simulink model "mariner_sim"  (R2018b)
settings: Solver=ode1  StartTime=0.0  StopTime=600  FixedStep=0.1  RelTol=1e-3
libraries: neural x408, simulink x2
(part 22 of 22)

== system mariner_sim/Plant/NN plant mariner (No delta_dot)/Layer 6/Delays 1 ==
  "p{6}" : Inport  PortDimensions=24
      mask Display: e = 0.06;c1 = [120 230 180]/255;c2 = ([120 230 180]+0)/(256+128);c3 = ([120 230 180]+128)/(256+128);patch([0 1 1 0],[0 0 1 1],c1);patch([0 1 1 1-e 1-e 0+e],[0 0 1 1-e 0+e 0+e],c2);patch([0 0 1 1-e 0+e 0+e],[0 1 1 1-e 1-e 0+e],c3);plot([0 1 1 0 0],[0 0 1 1 0]);
  mux : Mux  Inputs=1
      mask Display: e = 0.06;c1 = [120 150 230]/255;c2 = ([120 150 230]+0)/383;c3 = ([120 150 230]+128)/383;patch([0 1 1 0],[0 0 1 1],c1);patch([0 1 1 1-e 1-e 0+e],[0 0 1 1-e 0+e 0+e],c2);patch([0 0 1 1-e 0+e 0+e],[0 1 1 1-e 1-e 0+e],c3);plot([0 1 1 0 0],[0 0 1 1 0]);disp('Mux')
  "pd{6,5}" : Outport
      mask Display: e = 0.06;c1 = [120 230 180]/255;c2 = ([120 230 180]+0)/(256+128);c3 = ([120 230 180]+128)/(256+128);patch([0 1 1 0],[0 0 1 1],c1);patch([0 1 1 1-e 1-e 0+e],[0 0 1 1-e 0+e 0+e],c2);patch([0 0 1 1-e 0+e 0+e],[0 1 1 1-e 1-e 0+e],c3);plot([0 1 1 0 0],[0 0 1 1 0]);
  wires:
  mux/1 -> "pd{6,5}"/1
  "p{6}"/1 -> mux/1

== system mariner_sim/Plant/NN plant mariner (No delta_dot)/Layer 6/LW{6,5} ==
  "ad{6,5}" : Inport  PortDimensions=24
      mask Display: e = 0.06;c1 = [120 230 180]/255;c2 = ([120 230 180]+0)/(256+128);c3 = ([120 230 180]+128)/(256+128);patch([0 1 1 0],[0 0 1 1],c1);patch([0 1 1 1-e 1-e 0+e],[0 0 1 1-e 0+e 0+e],c2);patch([0 0 1 1-e 0+e 0+e],[0 1 1 1-e 1-e 0+e],c3);plot([0 1 1 0 0],[0 0 1 1 0]);
  "IW{6,5}(1,:)'" : Constant  Value=[3.2433598998004699938586814500496302571264095604419708251953125e-05;-0.00021746891264327707147911705742870935864630155265331268310546875;-6.2519957775104847519202777572644436077098362147808074951171875e-05;-0.0002151214461402426174514712631236079687369056046009063720703125;-7.72914603333618179491215638421408584690652787685394287109375e-05;9.8220947618367704444290733345468424886348657310009002685546875e-05;0.0001382930564768189885156701723900596334715373814105987548828125;0.0001645748510074347280458806341840727327507920563220977783203125;0.000268939822215103450930850925715276389382779598236083984375;6.2985224591444543651257148564326371342758648097515106201171875e-05;5.6838608479464312821347223014800675855440204031765460968017578125e-06;2.01845702968149283613487343647108218647190369665622711181640625e-05;0.0001676190564912218385930364750180388000444509088993072509765625;0.000135878965702839718705796645537020594929344952106475830078125;6.2205662182553546173113812045585291343741118907928466796875e-05;0.000111446864397163089934784940826517640743986703455448150634765625;-5.8634943766458073424502513149025872962738503701984882354736328125e-06;0.000112997310599974860162962586596080427625565789639949798583984375;2.846586362506669975656024840215962967704399488866329193115234375e-05;-0.0001710958953371501914571262137343410358880646526813507080078125;2.73394004824882604748857717336107953087775968015193939208984375e-05;-6.170901822294167123061914281834106077440083026885986328125e-05;8.1478519128559822736097839612767756989342160522937774658203125e-05;4.553422019458672740689630931143483394407667219638824462890625e-05]
      mask Display: e = 0.06;c1 = [120 150 230]/255;c2 = ([120 150 230]+0)/383;c3 = ([120 150 230]+128)/383;patch([0 1 1 0],[0 0 1 1],c1);patch([0 1 1 1-e 1-e 0+e],[0 0 1 1-e 0+e 0+e],c2);patch([0 0 1 1-e 0+e 0+e],[0 1 1 1-e 1-e 0+e],c3);plot([0 1 1 0 0],[0 0 1 1 0]);disp('weights');
  "IW{6,5}(2,:)'" : Constant  Value=[-0.000826529499500064574780966442091312273987568914890289306640625;-0.000642491212784880995172176465501934217172674834728240966796875;-0.00089601761422035386926709943367086452781222760677337646484375;0.0003640521562445046019167171902353175028110854327678680419921875;-0.0022597717662539919432351798178615354117937386035919189453125;-5.95161806487568421550858610569179063531919382512569427490234375e-05;-0.00025641552490142881758072856968055930337868630886077880859375;0.00080747921980977373397625473927519124117679893970489501953125;-0.00042040003190180522639474158808070569648407399654388427734375;0.0018262459479417773693110671473505135509185492992401123046875;-0.00146586650901986935424670122074530809186398983001708984375;7.8763674807919793123371643428498600769671611487865447998046875e-05;-0.00010991751878111353829710339358172177526284940540790557861328125;-0.00036678182453456676000158598327516301651485264301300048828125;-0.0003171821049869377631517941562577789227361790835857391357421875;0.000251068945369483233036322911146953629213385283946990966796875;-0.001212130785092036151795458209790012915618717670440673828125;0.000947577323859999267989528970446144739980809390544891357421875;0.00052599882450631301085419710972246321034617722034454345703125;-0.00081217642806952791527386192882431714679114520549774169921875;0.0047275051808355512961146160932912607677280902862548828125;-0.000635378248235334550965414113221640945994295179843902587890625;9.64182414439658107448150037299683390301652252674102783203125e-05;0.0001731850016870155610677894930660158934188075363636016845703125]
      mask Display: e = 0.06;c1 = [120 150 230]/255;c2 = ([120 150 230]+0)/383;c3 = ([120 150 230]+128)/383;patch([0 1 1 0],[0 0 1 1],c1);patch([0 1 1 1-e 1-e 0+e],[0 0 1 1-e 0+e 0+e],c2);patch([0 0 1 1-e 0+e 0+e],[0 1 1 1-e 1-e 0+e],c3);plot([0 1 1 0 0],[0 0 1 1 0]);disp('weights');
  "IW{6,5}(3,:)'" : Constant  Value=[2.46152644631382654040636925873997142844018526375293731689453125e-05;-2.563158103268046409013714015401319556985981762409210205078125e-05;1.19444456304550761520551216410268580148112960159778594970703125e-05;-3.8165061632398022094248002389349494478665292263031005859375e-05;3.2095720426049420353174779219074252978316508233547210693359375e-05;2.005335334908526424726842030121787274765665642917156219482421875e-05;4.76339293072544701685040735572584935653139837086200714111328125e-05;1.7604738734322618212528588355070269244606606662273406982421875e-05;6.1921630995887057030864497608746432888437993824481964111328125e-05;-2.677483879698117457388885365165975827039801515638828277587890625e-05;2.65402830536713558421020586752803183117066510021686553955078125e-05;6.980146402722020059004696956872493274204316549003124237060546875e-06;4.91862369857580910268747553804047356607043184340000152587890625e-05;9.398121921791441398127096851222717077689594589173793792724609375e-06;2.849932108961100444741686155136761726680560968816280364990234375e-05;2.474611348555533069906893495204514010765706188976764678955078125e-05;3.89805031900851425646047088147128079071990214288234710693359375e-05;-7.06469847394216254009291500182143863639794290065765380859375e-07;1.40147477682385900184768023901682454379624687135219573974609375e-05;-9.1741821131806661920350676187041472076089121401309967041015625e-06;-0.00012599257486806556753482222443807359013590030372142791748046875;7.964410532433889255391097627967411654026363976299762725830078125e-06;2.9571704172556262228167833772118910928838886320590972900390625e-05;-5.5995289024227002996621053998449468735998379997909069061279296875e-06]
      mask Display: e = 0.06;c1 = [120 150 230]/255;c2 = ([120 150 230]+0)/383;c3 = ([120 150 230]+128)/383;patch([0 1 1 0],[0 0 1 1],c1);patch([0 1 1 1-e 1-e 0+e],[0 0 1 1-e 0+e 0+e],c2);patch([0 0 1 1-e 0+e 0+e],[0 1 1 1-e 1-e 0+e],c3);plot([0 1 1 0 0],[0 0 1 1 0]);disp('weights');
  "IW{6,5}(4,:)'" : Constant  Value=[-0.1046999224485727630895581796721671707928180694580078125;-0.214859862140896529236755441161221824586391448974609375;-0.11414394274893570335738246512846671976149082183837890625;-0.193735966562724792883187774350517429411411285400390625;-0.1777661283319564855531780267483554780483245849609375;-0.406317254503526459341600229890900664031505584716796875;0.09130499074981761331581964213910396210849285125732421875;-0.08355202175896110639019553900652681477367877960205078125;0.004607169690688232670250368272490959498099982738494873046875;0.11331833976123040219619042545673437416553497314453125;0.12349327484238233065827472501041484065353870391845703125;-0.09737098152361088609918482461580424569547176361083984375;-0.172392956306251454723366123289451934397220611572265625;-0.05354406813646846174936655415876884944736957550048828125;0.0788347063873013897961072871112264692783355712890625;0.131548859513590021830253817824996076524257659912109375;0.258288818657371466169792029177187941968441009521484375;-0.3513774626571934955876486128545366227626800537109375;0.1285503858247094288724809985069441609084606170654296875;0.1822954729789078853752215536587755195796489715576171875;-0.05059362603293506011059577076593996025621891021728515625;0.1611838123398981748035652117323479615151882171630859375;-0.001358270969995178760469922707443402032367885112762451171875;0.1691231424475345967994854845528607256710529327392578125]
      mask Display: e = 0.06;c1 = [120 150 230]/255;c2 = ([120 150 230]+0)/383;c3 = ([120 150 230]+128)/383;patch([0 1 1 0],[0 0 1 1],c1);patch([0 1 1 1-e 1-e 0+e],[0 0 1 1-e 0+e 0+e],c2);patch([0 0 1 1-e 0+e 0+e],[0 1 1 1-e 1-e 0+e],c3);plot([0 1 1 0 0],[0 0 1 1 0]);disp('weights');
  "IW{6,5}(5,:)'" : Constant  Value=[-0.261050291944736445604036134682246483862400054931640625;0.21688530390838633987726780105731450021266937255859375;-0.0263686731508492311348845760221593081951141357421875;-0.0783502653405710181022669758021947927772998809814453125;-0.0574573045503896373542573883241857402026653289794921875;-0.02833691747677068162314384380806586705148220062255859375;0.306787389727579518083899756675236858427524566650390625;0.4115796583411033271460155447130091488361358642578125;-0.0884904419428817756720917486745747737586498260498046875;-0.04625755795249515689437913579240557737648487091064453125;-0.01312950851618376220397710341103447717614471912384033203125;0.148726783593528200100308822584338486194610595703125;-0.24354178610612653432809793230262584984302520751953125;0.2624174384097830436957110578077845275402069091796875;0.480136430526202584445627508102916181087493896484375;-0.3441908584282888927674548540380783379077911376953125;-0.145810822380717741708622270380146801471710205078125;0.307466536601382178783836707225418649613857269287109375;-0.1708275816058468787872470784350298345088958740234375;-0.22206736034940333102127851816476322710514068603515625;0.05136313987499152577953509535291232168674468994140625;0.0226850580484755093291227012741728685796260833740234375;-0.50394671901843557382250082810060121119022369384765625;-0.1788429832334376412550369650489301420748233795166015625]
      mask Display: e = 0.06;c1 = [120 150 230]/255;c2 = ([120 150 230]+0)/383;c3 = ([120 150 230]+128)/383;patch([0 1 1 0],[0 0 1 1],c1);patch([0 1 1 1-e 1-e 0+e],[0 0 1 1-e 0+e 0+e],c2);patch([0 0 1 1-e 0+e 0+e],[0 1 1 1-e 1-e 0+e],c3);plot([0 1 1 0 0],[0 0 1 1 0]);disp('weights');
  "IW{6,5}(6,:)'" : Constant  Value=[-8.3873490168356670273162867257354946559644304215908050537109375e-05;0.00147502001895182498214520450119380257092416286468505859375;0.000330261437779736277860209714418715520878322422504425048828125;0.00133625764264578878078026935583011436392553150653839111328125;0.00085914790987545578727913042627051254385150969028472900390625;-0.000567433998010235108970522599491914661484770476818084716796875;-0.0010907273517562336186126348280822639935649931430816650390625;-0.00133779757933903263762698276906348837655968964099884033203125;-0.00234554091843410493500865499072460806928575038909912109375;-0.0001144305367251422498632573709897997105144895613193511962890625;0.0003636845135138208986481933582268766258493997156620025634765625;-2.0497064683987363986790442016427959970314987003803253173828125e-05;-0.0013673893877836052444807446448749033152125775814056396484375;-0.00079367129654968858465391434720004326663911342620849609375;-0.000418521036158354671312398220806016979622654616832733154296875;-0.00104356258505614442159969978973776960629038512706756591796875;-0.000101142753841237495091541498393183928783400915563106536865234375;-0.00091411335818792249958975038026665060897357761859893798828125;-0.000743367293182789989035297306685379226109944283962249755859375;0.000889863084029751433452759545872368107666261494159698486328125;0.000803295392184018319271798791447736221016384661197662353515625;0.0004381772186861732716785244878821004022029228508472442626953125;-0.00147945223686744516990165809744439684436656534671783447265625;-0.0002851975628954128987209426515647692212951369583606719970703125]
      mask Display: e = 0.06;c1 = [120 150 230]/255;c2 = ([120 150 230]+0)/383;c3 = ([120 150 230]+128)/383;patch([0 1 1 0],[0 0 1 1],c1);patch([0 1 1 1-e 1-e 0+e],[0 0 1 1-e 0+e 0+e],c2);patch([0 0 1 1-e 0+e 0+e],[0 1 1 1-e 1-e 0+e],c3);plot([0 1 1 0 0],[0 0 1 1 0]);disp('weights');
  Mux : Mux  Inputs=6
      mask Display: e = 0.06;c1 = [120 150 230]/255;c2 = ([120 150 230]+0)/383;c3 = ([120 150 230]+128)/383;patch([0 1 1 0],[0 0 1 1],c1);patch([0 1 1 1-e 1-e 0+e],[0 0 1 1-e 0+e 0+e],c2);patch([0 0 1 1-e 0+e 0+e],[0 1 1 1-e 1-e 0+e],c3);plot([0 1 1 0 0],[0 0 1 1 0]);disp('Mux');
  dotprod{1..6} (6 alike) : neural/Weight Functions/dotprod
  "lz{6,5}" : Outport
      mask Display: e = 0.06;c1 = [120 230 180]/255;c2 = ([120 230 180]+0)/(256+128);c3 = ([120 230 180]+128)/(256+128);patch([0 1 1 0],[0 0 1 1],c1);patch([0 1 1 1-e 1-e 0+e],[0 0 1 1-e 0+e 0+e],c2);patch([0 0 1 1-e 0+e 0+e],[0 1 1 1-e 1-e 0+e],c3);plot([0 1 1 0 0],[0 0 1 1 0]);
  wires:
  Mux/1 -> "lz{6,5}"/1
  dotprod6/1 -> Mux/6
  "IW{6,5}(6,:)'"/1 -> dotprod6/1
  dotprod5/1 -> Mux/5
  "IW{6,5}(5,:)'"/1 -> dotprod5/1
  dotprod4/1 -> Mux/4
  "IW{6,5}(4,:)'"/1 -> dotprod4/1
  dotprod3/1 -> Mux/3
  "IW{6,5}(3,:)'"/1 -> dotprod3/1
  dotprod2/1 -> Mux/2
  "IW{6,5}(2,:)'"/1 -> dotprod2/1
  dotprod1/1 -> Mux/1
  "ad{6,5}"/1 -> dotprod6/2, dotprod5/2, dotprod4/2, dotprod3/2, dotprod2/2, dotprod1/2
  "IW{6,5}(1,:)'"/1 -> dotprod1/1

== matlab function mariner_sim/MATLAB Function1 ==
  data: xdot input; xnext output; x input; h input
function xnext = euler2(xdot,x,h)
% EULER2  Integrate a system of ordinary differential equations using 
%	  Euler's 2nd-order method.
%
% xnext = euler2(xdot,x,h)
%
% xdot  - dx/dt(k) = f(x(k)
% x     - x(k)
% xnext - x(k+1)
% h     - step size
%
% Author:   Thor I. Fossen
% Date:     14th June 2001
% Revisions: 

xnext = x + h*xdot;

== matlab function mariner_sim/MATLAB Function ==
  data: x input; xdot output; ui input
function xdot   = mariner(x,ui)
% [xdot,U] = mariner(x,ui) returns the speed U in m/s (optionally) and the 
% time derivative of the state vector: x = [ u v r x y psi delta n ]'  for
% the Mariner class vessel L = 160.93 m, where
%
% u     = pertubed surge velocity about Uo (m/s)
% v     = pertubed sway velocity about zero (m/s)
% r     = pertubed yaw velocity about zero (rad/s)
% x     = position in x-direction (m)
% y     = position in y-direction (m)
% psi   = pertubed yaw angle about zero (rad)
% delta = actual rudder angle (rad)
%
% The inputs are :
% 
% ui    = commanded rudder angle (rad)
% U0    = nominal speed (optionally). Default value is U0 = 7.7175 m/s = 15 knots.
%
% Reference: M.S. Chislett and J. Stroem-Tejsen (1965). Planar Motion Mechanism Tests 
%            and Full-Scale Steering and Maneuvering Predictions for a Mariner Class Vessel,
%            Technical Report Hy-5, Hydro- and Aerodynamics Laboratory, Lyngby, Denmark.
% 
% Author:    Trygve Lauvdal
% Date:      12th May 1994
% Revisions: 19th July 2001 (Thor I. Fossen): added input/ouput U0 and U, changed order of x-vector
%            20th July 2001 (Thor I. Fossen): replaced inertia matrix with correct values
%            11th July 2003 (Thor I. Fossen): max rudder is changed from 30 deg to 40
%                            deg to satisfy IMO regulations for 35 deg rudder execute

% Check of input and state dimensions
if (length(x)  ~= 7),error('x-vector must have dimension 7 !'); end
if (length(ui) ~= 1),error('ui must be a scalar input!'); end
%if nargin==2, U0 = 7.7175; end

U0 = 7.7175;

% Normalization variables
L = 160.93;
U = sqrt((U0 + x(1))^2 + x(2)^2);

% Non-dimensional states and inputs
delta_c = -ui;   % delta_c = -ui such that positive delta_c -> positive r

u     = x(1)/U;   
v     = x(2)/U;  
r     = x(3)*L/U; 
psi   = x(6); 
delta = x(7); 

% Parameters, hydrodynamic derivatives and main dimensions
delta_max  = 40;           % max rudder angle      (deg)
Ddelta_max = 5;            % max rudder derivative (deg/s)

m  = 798e-5;
Iz = 39.2e-5;
xG = -0.023;

Xudot =  -42e-5;   Yvdot =  -748e-5;   Nvdot = 4.646e-5;
Xu    = -184e-5;   Yrdot =-9.354e-5;   Nrdot = -43.8e-5;
Xuu   = -110e-5;   Yv    = -1160e-5;   Nv    =  -264e-5;
Xuuu  = -215e-5;   Yr    =  -499e-5;   Nr    =  -166e-5;
Xvv   = -899e-5;   Yvvv  = -8078e-5;   Nvvv  =  1636e-5;
Xrr   =   18e-5;   Yvvr  = 15356e-5;   Nvvr  = -5483e-5;
Xdd   =  -95e-5;   Yvu   = -1160e-5;   Nvu   =  -264e-5;
Xudd  = -190e-5;   Yru   =  -499e-5;   Nru   =  -166e-5;
Xrv   =  798e-5;   Yd    =   278e-5;   Nd    =  -139e-5;
Xvd   =   93e-5;   Yddd  =   -90e-5;   Nddd  =    45e-5;
Xuvd  =   93e-5;   Yud   =   556e-5;   Nud   =  -278e-5;
                   Yuud  =   278e-5;   Nuud  =  -139e-5;
                   Yvdd  =    -4e-5;   Nvdd  =    13e-5;
                   Yvvd  =  1190e-5;   Nvvd  =  -489e-5;
                   Y0    =    -4e-5;   N0    =     3e-5;
                   Y0u   =    -8e-5;   N0u   =     6e-5;
                   Y0uu  =    -4e-5;   N0uu  =     3e-5;

% Masses and moments of inertia
m11 = m-Xudot;
m22 = m-Yvdot;
m23 = m*xG-Yrdot;
m32 = m*xG-Nvdot;
m33 = Iz-Nrdot;

% Rudder saturation and dynamics
if abs(delta_c) >= delta_max*pi/180,
   delta_c = sign(delta_c)*delta_max*pi/180;
end
delta_dot = delta_c - delta;
if abs(delta_dot) >= Ddelta_max*pi/180,
   delta_dot = sign(delta_dot)*Ddelta_max*pi/180;
end

% Forces and moments
X = Xu*u + Xuu*u^2 + Xuuu*u^3 + Xvv*v^2 + Xrr*r^2 + Xrv*r*v + Xdd*delta^2 +...
    Xudd*u*delta^2 + Xvd*v*delta + Xuvd*u*v*delta;

Y = Yv*v + Yr*r + Yvvv*v^3 + Yvvr*v^2*r + Yvu*v*u + Yru*r*u + Yd*delta + ...
    Yddd*delta^3 + Yud*u*delta + Yuud*u^2*delta + Yvdd*v*delta^2 + ...
    Yvvd*v^2*delta + (Y0 + Y0u*u + Y0uu*u^2);

N = Nv*v + Nr*r + Nvvv*v^3 + Nvvr*v^2*r + Nvu*v*u + Nru*r*u + Nd*delta + ...
    Nddd*delta^3 + Nud*u*delta + Nuud*u^2*delta + Nvdd*v*delta^2 + ...
    Nvvd*v^2*delta + (N0 + N0u*u + N0uu*u^2);

% Dimensional state derivative
detM22 = m22*m33-m23*m32;

xdot = [           X*(U^2/L)/m11
        -(-m33*Y+m23*N)*(U^2/L)/detM22
         (-m32*Y+m22*N)*(U^2/L^2)/detM22
           (cos(psi)*(U0/U+u)-sin(psi)*v)*U
           (sin(psi)*(U0/U+u)+cos(psi)*v)*U  
                    r*(U/L)
                    delta_dot                  ];

== stateflow chart mariner_sim/mariner ==
  settings: updateMethod=CONTINUOUS
  state mariner
    %% initialize values when entry
    en:
    L = 160.93;
    m = 798*10^-5;
    xG = -0.023;
    Iz = 39.2*10^-5;
    Xudot =  -42e-5;  Yvdot =  -748e-5;  Nvdot = 4.646e-5;
    Xu  = -184e-5;   Yrdot =-9.354e-5;   Nrdot = -43.8e-5;
    Xuu = -110e-5;   Yv = -1160e-5;   Nv =  -264e-5;
    Xuuu = -215e-5;   Yr =  -499e-5;   Nr =  -166e-5;
    Xvv = -899e-5;   Yvvv = -8078e-5;   Nvvv =  1636e-5;
    Xrr =   18e-5;   Yvvr = 15356e-5;   Nvvr = -5483e-5;
    Xdd =  -95e-5;   Yvu = -1160e-5;   Nvu =  -264e-5;
    Xudd = -190e-5;   Yru =  -499e-5;   Nru =  -166e-5;
    Xrv =  798e-5;   Yd  =   278e-5;   Nd =  -139e-5;
    Xvd =   93e-5;   Yddd  =   -90e-5;   Nddd =    45e-5;
    Xuvd =   93e-5;   Yud = 556e-5;   Nud =  -278e-5;
    Yuud =   278e-5;   Nuud  =  -139e-5;
    Yvdd  =    -4e-5;   Nvdd  = 13e-5;
    Yvvd  =  1190e-5;   Nvvd  = -489e-5;
    Y0 = -4e-5;   N0 =  3e-5;
    Y0u  =  -8e-5;   N0u = 6e-5;
    Y0uu =  -4e-5;   N0uu  =  3e-5;
    m11 = 798*10^-5 - (-42e-5);
    m22 = 798*10^-5 - ( -748e-5);
    m23 = 798*10^-5 * -0.023 - (-9.354e-5);
    m32 = 798*10^-5 * -0.023 - 4.646e-5;
    m33 = 39.2*10^-5 -  (-43.8e-5);
    %detM22 = m22*m33-m23*m32;
    %detM22 = ((798*10^-5 - ( -748e-5))*(39.2*10^-5 -  (-43.8e-5)) - (798*10^-5 * -0.023 - (-9.354e-5))*(798*10^-5 * -0.023 - 4.646e-5));
    delta_max = 40;
    Ddelta_max = 5;
    % u
    %Executing updates of system during simulation
    du:
    %delta_c = min(max(-ui,-delta_max*pi/180),delta_max*pi/180) ;
    %U = (sqrt((ui + u)^2 + v^2));
    %delta_do = (-ui - delta);
    %X = Xu*u/(sqrt((ui + u)^2 + v^2)) + Xuu*(u/(sqrt((ui + u)^2 + v^2)))^2 + Xuuu*(u/(sqrt((ui + u)^2 + v^2)))^3 + Xvv*(v/(sqrt((ui + u)^2 + v^2)))^2 + Xrr*(r*L/(sqrt((ui + u)^2 + v^2)))^2 + Xrv*(r*L/(sqrt((ui + u)^2 + v^2)))*(v/(sqrt((ui + u)^2 + v^2))) + Xdd*delta^2 +Xudd*(u/(sqrt((ui + u)^2 + v^2)))*delta^2 + Xvd*(v/(sqrt((ui + u)^2 + v^2)))*delta + Xuvd*(u/(sqrt((ui + u)^2 + v^2)))*(v/(sqrt((ui + u)^2 + v^2)))*delta;
    %Y = Yv*v + Yr*r + Yvvv*v^3 + Yvvr*v^2*r + Yvu*v*u + Yru*r*u + Yd*delta + Yddd*delta^3 + Yud*u*delta + Yuud*u^2*delta + Yvdd*v*delta^2 + Yvvd*v^2*delta + (Y0 + Y0u*u + Y0uu*u^2);
    %N = Nv*v + Nr*r + Nvvv*v^3 + Nvvr*v^2*r + Nvu*v*u + Nru*r*u + Nd*delta + Nddd*delta^3 + Nud*u*delta + Nuud*u^2*delta + Nvdd*v*delta^2 + Nvvd*v^2*delta + (N0 + N0u*u + N0uu*u^2);
    u_dot = (Xu*(u/(sqrt((ui + u)^2 + v^2))) + Xuu*(u/(sqrt((ui + u)^2 + v^2)))^2 + Xuuu*(u/(sqrt((ui + u)^2 + v^2)))^3 + Xvv*(v/(sqrt((ui + u)^2 + v^2)))^2 + Xrr*(r*L/(sqrt((ui + u)^2 + v^2)))^2 + Xrv*(r*L/(sqrt((ui + u)^2 + v^2)))*(v/(sqrt((ui + u)^2 + v^2))) + Xdd*delta^2 +Xudd*(u/(sqrt((ui + u)^2 + v^2)))*delta^2 + Xvd*(v/(sqrt((ui + u)^2 + v^2)))*delta + Xuvd*(u/(sqrt((ui + u)^2 + v^2)))*(v/(sqrt((ui + u)^2 + v^2)))*delta)*((sqrt((ui + u)^2 + v^2))^2 /L)/(798*10^-5 - (-42e-5));
    v_dot =  -(-(39.2*10^-5 -  (-43.8e-5))*(Yv*(v/(sqrt((ui + u)^2 + v^2))) + Yr*(r*L/(sqrt((ui + u)^2 + v^2))) + Yvvv*(v/(sqrt((ui + u)^2 + v^2)))^3 + Yvvr*(v/(sqrt((ui + u)^2 + v^2)))^2 * (r*L/(sqrt((ui + u)^2 + v^2))) + Yvu*(v/(sqrt((ui + u)^2 + v^2)))*(u/(sqrt((ui + u)^2 + v^2))) + Yru*(r*L/(sqrt((ui + u)^2 + v^2)))*(u/(sqrt((ui + u)^2 + v^2))) + Yd*delta + Yddd*delta^3 + Yud*(u/(sqrt((ui + u)^2 + v^2)))*delta + Yuud*(u/(sqrt((ui + u)^2 + v^2)))^2*delta + Yvdd*(v/(sqrt((ui + u)^2 + v^2)))*delta^2 + Yvvd*(v/(sqrt((ui + u)^2 + v^2)))^2*delta + (Y0 + Y0u*(u/(sqrt((ui + u)^2 + v^2))) + Y0uu*(u/(sqrt((ui + u)^2 + v^2)))^2))+(798*10^-5 * -0.023 - (-9.354e-5))*(Nv*(v/(sqrt((ui + u)^2 + v^2))) + Nr*(r*L/(sqrt((ui + u)^2 + v^2))) + Nvvv*(v/(sqrt((ui + u)^2 + v^2)))^3 + Nvvr*(v/(sqrt((ui + u)^2 + v^2)))^2*(r*L/(sqrt((ui + u)^2 + v^2))) + Nvu*(v/(sqrt((ui + u)^2 + v^2)))*(u/(sqrt((ui + u)^2 + v^2))) + Nru*(r*L/(sqrt((ui + u)^2 + v^2)))*(u/(sqrt((ui + u)^2 + v^2))) + Nd*delta + Nddd*delta^3 + Nud*(u/(sqrt((ui + u)^2 + v^2)))*delta + Nuud*(u/(sqrt((ui + u)^2 + v^2)))^2*delta + Nvdd*(v/(sqrt((ui + u)^2 + v^2)))*delta^2 + Nvvd*v^2*delta + (N0 + N0u*u + N0uu*u^2)))*((sqrt((ui + u)^2 + v^2))^2/L)/((798*10^-5 - ( -748e-5))*(39.2*10^-5 -  (-43.8e-5)) - (798*10^-5 * -0.023 - (-9.354e-5))*(798*10^-5 * -0.023 - 4.646e-5)) ;
    r_dot = (-(798*10^-5 * -0.023 - 4.646e-5)*(Yv*(v/(sqrt((ui + u)^2 + v^2))) + Yr*(r*L/(sqrt((ui + u)^2 + v^2))) + Yvvv*(v/(sqrt((ui + u)^2 + v^2)))^3 + Yvvr*(v/(sqrt((ui + u)^2 + v^2)))^2*(r*L/(sqrt((ui + u)^2 + v^2))) + Yvu*(v/(sqrt((ui + u)^2 + v^2)))*(u/(sqrt((ui + u)^2 + v^2))) + Yru*(r*L/(sqrt((ui + u)^2 + v^2)))*(u/(sqrt((ui + u)^2 + v^2))) + Yd*delta + Yddd*delta^3 + Yud*(u/(sqrt((ui + u)^2 + v^2)))*delta + Yuud*(u/(sqrt((ui + u)^2 + v^2)))^2*delta + Yvdd*(v/(sqrt((ui + u)^2 + v^2)))*delta^2 + Yvvd*(v/(sqrt((ui + u)^2 + v^2)))^2*delta + (Y0 + Y0u*(u/(sqrt((ui + u)^2 + v^2))) + Y0uu*(u/(sqrt((ui + u)^2 + v^2)))^2))+(798*10^-5 - ( -748e-5))*(Nv*(v/(sqrt((ui + u)^2 + v^2))) + Nr*(r*L/(sqrt((ui + u)^2 + v^2))) + Nvvv*(v/(sqrt((ui + u)^2 + v^2)))^3 + Nvvr*(v/(sqrt((ui + u)^2 + v^2)))^2*(r*L/(sqrt((ui + u)^2 + v^2))) + Nvu*(v/(sqrt((ui + u)^2 + v^2)))*(u/(sqrt((ui + u)^2 + v^2))) + Nru*(r*L/(sqrt((ui + u)^2 + v^2)))*(u/(sqrt((ui + u)^2 + v^2))) + Nd*delta + Nddd*delta^3 + Nud*(u/(sqrt((ui + u)^2 + v^2)))*delta + Nuud*(u/(sqrt((ui + u)^2 + v^2)))^2*delta + Nvdd*(v/(sqrt((ui + u)^2 + v^2)))*delta^2 + Nvvd*(v/(sqrt((ui + u)^2 + v^2)))^2*delta + (N0 + N0u*(u/(sqrt((ui + u)^2 + v^2))) + N0uu*(u/(sqrt((ui + u)^2 + v^2)))^2)))*((sqrt((ui + u)^2 + v^2))^2/L^2)/((798*10^-5 - ( -748e-5))*(39.2*10^-5 -  (-43.8e-5)) - (798*10^-5 * -0.023 - (-9.354e-5))*(798*10^-5 * -0.023 - 4.646e-5)) ;
    x_dot = (cos(psi)*(U0/(sqrt((ui + u)^2 + v^2))+(u/(sqrt((ui + u)^2 + v^2))))-sin(psi)*(v/(sqrt((ui + u)^2 + v^2))))*(sqrt((ui + u)^2 + v^2)) ;
    y_dot = (sin(psi)*(U0/(sqrt((ui + u)^2 + v^2))+(u/(sqrt((ui + u)^2 + v^2))))+cos(psi)*(v/(sqrt((ui + u)^2 + v^2))))*(sqrt((ui + u)^2 + v^2)) ;
    psi_dot = (r*L/(sqrt((ui + u)^2 + v^2)))*((sqrt((ui + u)^2 + v^2))/L);
    delta_dot = min(max(((min(max(-ui,-delta_max*pi/180),delta_max*pi/180)) - delta),-Ddelta_max*pi/180),Ddelta_max*pi/180) ;
    %% OUTPUTS
    u_out = u;
    v_out = v;
    r_out = r;
    x_out = x;
    y_out = y;
    psi_out = psi;
    delta_out = delta;
  (default) -> ? [order 1]
  (default) -> mariner [order 1] : {u = 0.01;
      | v = 0.01;
      | r = 0.01;
      | x = 0.01;
      | y = 0.01;
      | psi = 0.01;
      | delta = 0.01;}
  data: u_out output; v_out output; u local; ui input; v local; Nvdot local double; Iz local double; L local double; Yvdot local double; xG local double; m local double; Xudot local double; Xuu local double; Yv local double; Xuuu local double; Nrdot local double; Nv local double; Yr local double; Yrdot local double; Xu local double; Nr local double; Xrr local double; Xdd local double; Yvvv local double; Yvu local double; Nvvv local double; Yvvr local double; Nvvr local double; Xvv local double; Xvd local double; Yru local double; Nd local double; Nvu local double; Xudd local double; Nru local double; Yd local double; Xrv local double; Nvdd local double; Yud local double; Yuud local double; Xuvd local double; Yvdd local double; Nud local double; Nuud local double; Yddd local double; Nddd local double; Y0uu local double; N0uu local double; N0 local double; N0u local double; Y0 local double; Yvvd local double; Nvvd local double; Y0u local double; m11 local double; m32 local double; m22 local double; m23 local double; m33 local double; U0 input; r_out output; r local; psi local; x local; y local; delta local; Ddelta_max local double; delta_max local double; N local double; x_out output; y_out output; psi_out output double; delta_out output
  data u settings: updateMethod=SF_CONTINUOUS_TIME_DATA
  data v settings: updateMethod=SF_CONTINUOUS_TIME_DATA
  data r settings: updateMethod=SF_CONTINUOUS_TIME_DATA
  data psi settings: updateMethod=SF_CONTINUOUS_TIME_DATA
  data x settings: updateMethod=SF_CONTINUOUS_TIME_DATA
  data y settings: updateMethod=SF_CONTINUOUS_TIME_DATA
  data delta settings: updateMethod=SF_CONTINUOUS_TIME_DATA

== matlab function mariner_sim/Plant/delta_dot ==
  data: u input; y output
function y = fcn(u)

% Parameters, hydrodynamic derivatives and main dimensions
delta_max  = 40;           % max rudder angle      (deg)
Ddelta_max = 5;            % max rudder derivative (deg/s)

% Non-dimensional states and inputs
delta_c = -u(8);   % delta_c = -ui such that positive delta_c -> positive 

% Rudder saturation and dynamics
if abs(delta_c) >= delta_max*pi/180
   delta_c = sign(delta_c)*delta_max*pi/180;
end
delta_dot = delta_c - u(8);
if abs(delta_dot) >= Ddelta_max*pi/180
   delta_dot = sign(delta_dot)*Ddelta_max*pi/180;
end
y = delta_dot;

== matlab function mariner_sim/Plant/normalize ==
  data: u input; y output
function y = fcn(u)
u_max = 0; u_min = -0.0186;
v_max = 0.1215; v_min = -0.1642;
r_max = 0.0028; r_min = -0.0019;
x_max = 4.6298e3; x_min = 0;
y_max = 469.4378; y_min = -305.1732;
psi_max = 0.1275; psi_min = -0.0850;
delta_max = 0.0839; delta_min = -0.0764;
cont_max = 0.0895; cont_min = -0.0879;
y = zeros(8,1);
y(1) = (u(1) - u_max)/(u_max-u_min);
y(2) = (u(2) - v_max)/(v_max-v_min);
y(3) = (u(3) - r_max)/(r_max-r_min);
y(4) = (u(4) - x_max)/(x_max-x_min);
y(5) = (u(5) - y_max)/(y_max-y_min);
y(6) = (u(6) - psi_max)/(psi_max-psi_min);
y(7) = (u(7) - delta_max)/(delta_max-delta_min);
y(8) = (u(8) - cont_max)/(cont_max - cont_min);

== matlab function mariner_sim/Plant/denormalize ==
  data: u input; y output
function y = fcn(u)
u_max = 1.19943-4; u_min = -4.6415e-04;
v_max = 0.0056; v_min = -0.0080;
r_max = 3.1583e-04; r_min = -1.9958e-04;
x_max = 7.7175; x_min = 7.6397;
y_max = 0.9653; y_min = -0.6235;
psi_max = 0.0029; psi_min = -0.0019;
%delta_max = 0.0873; delta_min = -0.0865;
y = zeros(6,1);
y(1) = u(1)*(u_max - u_min) + x_min;
y(2) = u(2)*(v_max - v_min) + y_min;
y(3) = u(3)*(r_max - r_min) + r_min;
y(4) = u(4)*(x_max - x_min) + x_min;
y(5) = u(5)*(y_max - y_min) + y_min;
y(6) = u(6)*(psi_max - psi_min) + psi_min;
%y(7) = u(1)*(u_max - u_min) + u_min;
